simulink model "model_no_heading_control"  (R2023b)
settings: Solver=VariableStepAuto  StartTime=0.0  StopTime=10.0  RelTol=1e-3
values from neighbouring files (symbols this model uses):
  turnrate_ref = 1    [get_heading_tf.m]
  turnrate_ref_start_time = 0.10    (= 0.1)    [get_heading_tf.m]
undefined symbols (not defined in the file or in its folder): acceleration_limit, alpha, D, gear, J, Kb, Ki, Ki_turnrate, Kp, Kp_turnrate, Kt, L, M, R, taud, transport_delay, Ts, turn_acc_limit, vel_ref, vel_ref_start_time, wheel_distance, wrad, wzi
settings Model: Creator=Gianluca  LastModifiedBy=simone

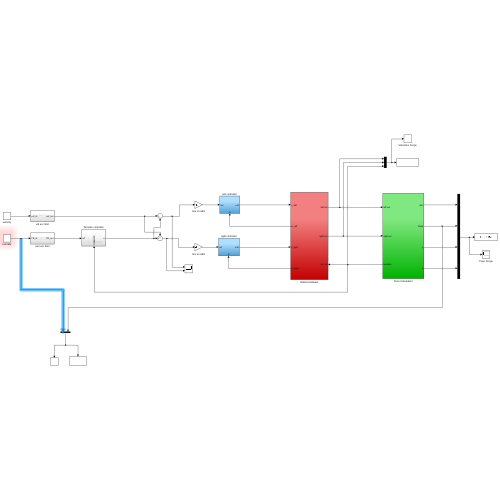
[thumbnail: Simulink's stored preview of the top-level diagram]
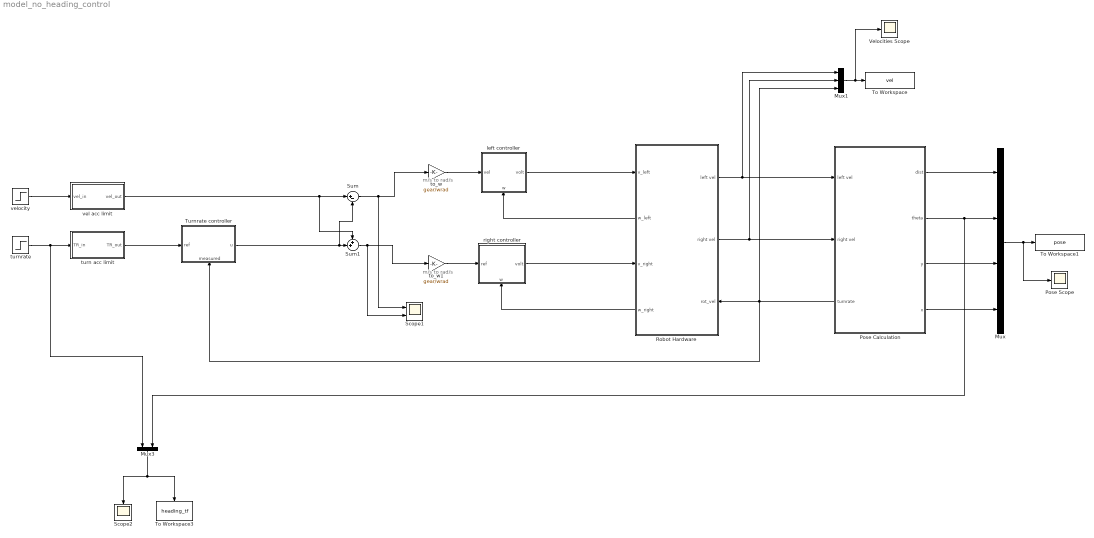
== system model_no_heading_control ==
  note: m/s to rad/s
  note: m/s to rad/s
  Mux : Mux
  Mux1 : Mux  Inputs=3
  Mux3 : Mux  Inputs=2
  Pose Calculation : Subsystem
      settings: PortSchema="{\"entries\":[{\"content\":{\"sides\":[{\"content\":{\"connectorIds\":[\"In1\",\"In2\",\"Out5\"]},\"type\":\"ConnectorPlacement.EquallySpacedRectSide\",\"uuid\":\"3bde791d-a2ac-4d13-a51a-30874ee8f75a\"},{\"content\":{\"connectorIds\":[\"Out1\",\"Out2\",\"Out3\",\"Out4\"],\"side\":\"RIGHT\"},\"type\":\"ConnectorPlacement.EquallySpacedRectSide\",\"uuid\":\"88ae4683-d3e7-483e-be55-3d26372f5fe2\"},{\"content\":{\"side\":\"TOP\"},\"type\":\"ConnectorPlacement.EquallySpacedRectSide\",\"uuid\":\"26752a72-f697-4de9-9dcd-1ca4cee0df39\"}]},\"type\":\"ConnectorPlacement.EquallySpacedConnector\",\"uuid\":\"d259c3e3-c5d7-42b6-881b-3a633aa969c6\"}],\"packageUris\":[\"http://schema.mathworks.com/mf0/Connector/R2020b\"],\"version\":\"1.0\"}"
  Pose Scope : Scope
  Robot Hardware : Subsystem
      settings: PortSchema="{\"entries\":[{\"content\":{\"sides\":[{\"content\":{\"connectorIds\":[\"In1\",\"Out3\",\"In2\",\"Out4\"]},\"type\":\"ConnectorPlacement.EquallySpacedRectSide\",\"uuid\":\"419fea77-f9ca-4e06-bea6-681a18650ab8\"},{\"content\":{\"connectorIds\":[\"Out1\",\"Out2\",\"In3\"],\"side\":\"RIGHT\"},\"type\":\"ConnectorPlacement.EquallySpacedRectSide\",\"uuid\":\"1629cad4-6101-470f-acc1-fad0cb327def\"},{\"content\":{\"side\":\"TOP\"},\"type\":\"ConnectorPlacement.EquallySpacedRectSide\",\"uuid\":\"70c90e71-c188-4b9c-b220-781da08827f9\"}]},\"type\":\"ConnectorPlacement.EquallySpacedConnector\",\"uuid\":\"ad56978f-143c-418e-863d-6c6f1f6f5d0c\"}],\"packageUris\":[\"http://schema.mathworks.com/mf0/Connector/R2020b\"],\"version\":\"1.0\"}"
  Scope1 : Scope  NumInputPorts=2
  Scope2 : Scope
  Sum : Sum  Inputs=|+-
  Sum1 : Sum  Inputs=++|
  To Workspace : ToWorkspace  VariableName=vel  SaveFormat=Timeseries  SampleTime=-1
  To Workspace1 : ToWorkspace  VariableName=pose  SaveFormat=Timeseries  SampleTime=-1
  To Workspace3 : ToWorkspace  VariableName=heading_tf  SaveFormat=Timeseries  SampleTime=-1
  Turnrate controller : Subsystem
      settings: PortSchema="{\"entries\":[{\"content\":{\"sides\":[{\"content\":{\"connectorIds\":[\"In1\"]},\"type\":\"ConnectorPlacement.EquallySpacedRectSide\",\"uuid\":\"3bde791d-a2ac-4d13-a51a-30874ee8f75a\"},{\"content\":{\"connectorIds\":[\"Out1\"],\"side\":\"RIGHT\"},\"type\":\"ConnectorPlacement.EquallySpacedRectSide\",\"uuid\":\"88ae4683-d3e7-483e-be55-3d26372f5fe2\"},{\"content\":{\"side\":\"TOP\"},\"type\":\"ConnectorPlacement.EquallySpacedRectSide\",\"uuid\":\"26752a72-f697-4de9-9dcd-1ca4cee0df39\"},{\"content\":{\"connectorIds\":[\"In2\"],\"side\":\"BOTTOM\"},\"type\":\"ConnectorPlacement.EquallySpacedRectSide\",\"uuid\":\"98a7b674-7c45-4a73-92a3-8750bdde1f36\"}]},\"type\":\"ConnectorPlacement.EquallySpacedConnector\",\"uuid\":\"d259c3e3-c5d7-42b6-881b-3a633aa969c6\"}],\"packageUris\":[\"http://schema.mathworks.com/mf0/Connector/R2020b\"],\"version\":\"1.0\"}"
  Velocities Scope : Scope
  left controller : Subsystem
      settings: PortSchema="{\"entries\":[{\"content\":{\"sides\":[{\"content\":{\"connectorIds\":[\"In1\"]},\"type\":\"ConnectorPlacement.EquallySpacedRectSide\",\"uuid\":\"3bde791d-a2ac-4d13-a51a-30874ee8f75a\"},{\"content\":{\"connectorIds\":[\"Out1\"],\"side\":\"RIGHT\"},\"type\":\"ConnectorPlacement.EquallySpacedRectSide\",\"uuid\":\"88ae4683-d3e7-483e-be55-3d26372f5fe2\"},{\"content\":{\"side\":\"TOP\"},\"type\":\"ConnectorPlacement.EquallySpacedRectSide\",\"uuid\":\"26752a72-f697-4de9-9dcd-1ca4cee0df39\"},{\"content\":{\"connectorIds\":[\"In2\"],\"side\":\"BOTTOM\"},\"type\":\"ConnectorPlacement.EquallySpacedRectSide\",\"uuid\":\"8837b86a-35cd-4679-9975-e69b760c287c\"}]},\"type\":\"ConnectorPlacement.EquallySpacedConnector\",\"uuid\":\"d259c3e3-c5d7-42b6-881b-3a633aa969c6\"}],\"packageUris\":[\"http://schema.mathworks.com/mf0/Connector/R2020b\"],\"version\":\"1.0\"}"
  right controller : Subsystem
      settings: PortSchema="{\"entries\":[{\"content\":{\"sides\":[{\"content\":{\"connectorIds\":[\"In1\"]},\"type\":\"ConnectorPlacement.EquallySpacedRectSide\",\"uuid\":\"3bde791d-a2ac-4d13-a51a-30874ee8f75a\"},{\"content\":{\"connectorIds\":[\"Out1\"],\"side\":\"RIGHT\"},\"type\":\"ConnectorPlacement.EquallySpacedRectSide\",\"uuid\":\"88ae4683-d3e7-483e-be55-3d26372f5fe2\"},{\"content\":{\"side\":\"TOP\"},\"type\":\"ConnectorPlacement.EquallySpacedRectSide\",\"uuid\":\"26752a72-f697-4de9-9dcd-1ca4cee0df39\"},{\"content\":{\"connectorIds\":[\"In2\"],\"side\":\"BOTTOM\"},\"type\":\"ConnectorPlacement.EquallySpacedRectSide\",\"uuid\":\"1adabdfb-f360-4bb8-8b57-8160c74899b3\"}]},\"type\":\"ConnectorPlacement.EquallySpacedConnector\",\"uuid\":\"d259c3e3-c5d7-42b6-881b-3a633aa969c6\"}],\"packageUris\":[\"http://schema.mathworks.com/mf0/Connector/R2020b\"],\"version\":\"1.0\"}"
  to_w : Gain  Gain=gear/wrad
  to_w1 : Gain  Gain=gear/wrad
  turn acc limit : Subsystem
  turnrate : Step  Time=turnrate_ref_start_time  After=turnrate_ref  SampleTime=0
  vel acc limit : Subsystem
  velocity : Step  Time=vel_ref_start_time  After=vel_ref  SampleTime=0
  wires:
  Sum/1 -> Scope1/1, to_w/1
  Sum1/1 -> Scope1/2, to_w1/1
  to_w/1 -> left controller/1(vel)
  to_w1/1 -> right controller/1(ref)
  Robot Hardware/4(w_right) -> right controller/2(w)
  right controller/1(volt) -> Robot Hardware/2(v_right)
  Robot Hardware/3(w_left) -> left controller/2(w)
  left controller/1(volt) -> Robot Hardware/1(v_left)
  Pose Calculation/5(turnrate) -> Turnrate controller/2(measured), Robot Hardware/3(rot_vel), Mux1/3
  Robot Hardware/2(right vel) -> Pose Calculation/2(right vel), Mux1/2
  Robot Hardware/1(left vel) -> Mux1/1, Pose Calculation/1(left vel)
  Mux/1 -> Pose Scope/1, To Workspace1/1
  Pose Calculation/3(y) -> Mux/3
  Pose Calculation/2(theta) -> Mux/2, Mux3/2
  Pose Calculation/1(dist) -> Mux/1
  Pose Calculation/4(x) -> Mux/4
  Mux1/1 -> Velocities Scope/1, To Workspace/1
  Turnrate controller/1(u) -> Sum/2, Sum1/2
  velocity/1 -> vel acc limit/1(vel_in)
  turnrate/1 -> Mux3/1, turn acc limit/1(TR_in)
  Mux3/1 -> To Workspace3/1, Scope2/1
  turn acc limit/1(TR_out) -> Turnrate controller/1(ref)
  vel acc limit/1(vel_out) -> Sum1/1, Sum/1

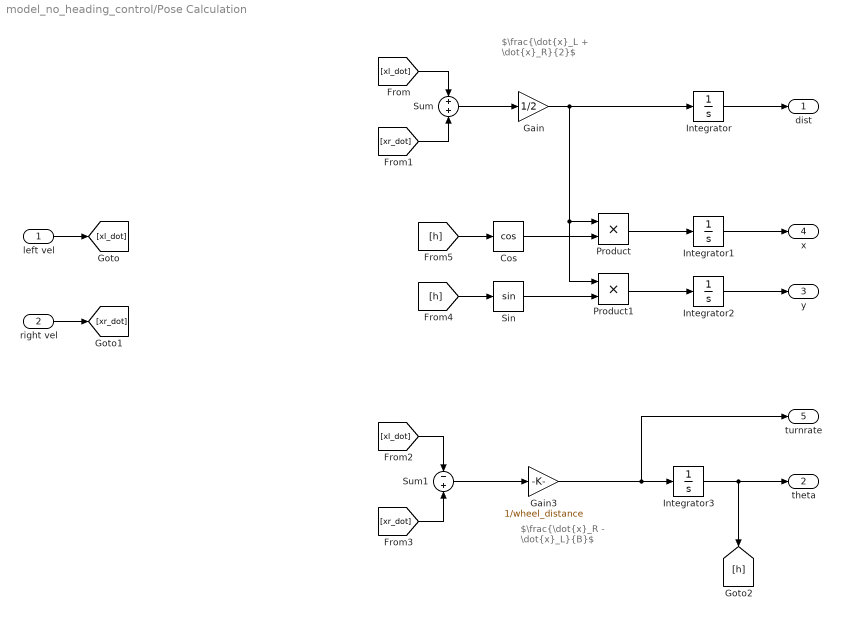
== system model_no_heading_control/Pose Calculation ==
  note: $\frac{\dot{x}_L + \dot{x}_R}{2}$
  note: $\frac{\dot{x}_R - \dot{x}_L}{B}$
  left vel : Inport
  right vel : Inport  Port=2
  Cos : Trigonometry  Operator=cos
  Gain : Gain  Gain=1/2
  Gain3 : Gain  Gain=1/wheel_distance
  Integrator{,1..3} (4 alike) : Integrator
  Product : Product
  Product1 : Product
  Sin : Trigonometry
  Sum : Sum  Inputs=+|+
  Sum1 : Sum  Inputs=-|+
  dist : Outport
  theta : Outport  Port=2
  y : Outport  Port=3
  x : Outport  Port=4
  turnrate : Outport  Port=5
  wires:
  Sum/1 -> Gain/1
  Gain/1 -> Integrator/1, Product/1, Product1/1
  Integrator/1 -> dist/1
  left vel/1 -> [xl_dot]
  right vel/1 -> [xr_dot]
  [xl_dot] -> Sum/1
  [xr_dot] -> Sum/2
  [xl_dot] -> Sum1/1
  [xr_dot] -> Sum1/2
  Gain3/1 -> turnrate/1, Integrator3/1
  Sum1/1 -> Gain3/1
  Integrator3/1 -> theta/1, [h]
  [h] -> Sin/1
  Integrator2/1 -> y/1
  Integrator1/1 -> x/1
  [h] -> Cos/1
  Sin/1 -> Product1/2
  Cos/1 -> Product/2
  Product1/1 -> Integrator2/1
  Product/1 -> Integrator1/1

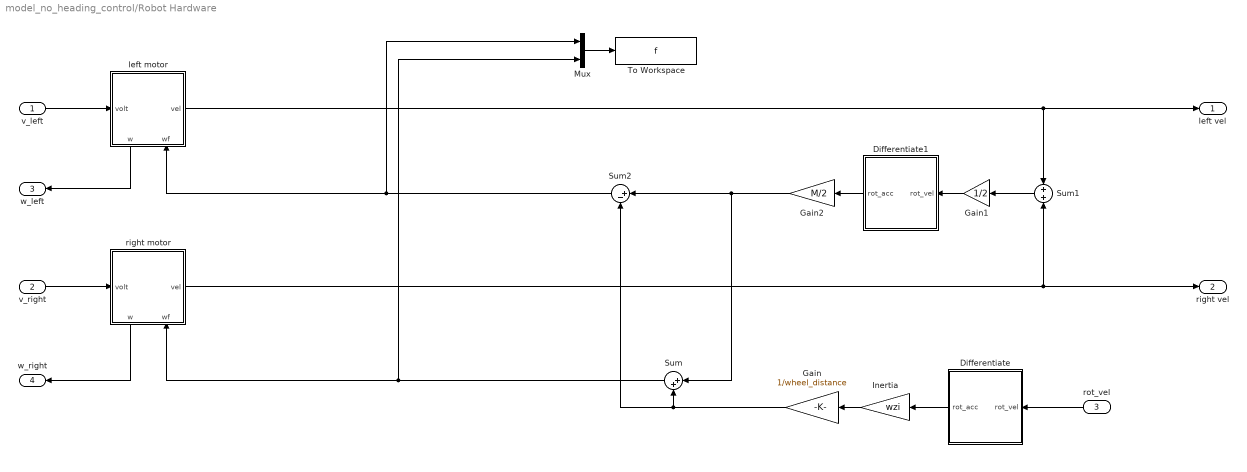
== system model_no_heading_control/Robot Hardware ==
  v_left : Inport
  v_right : Inport  Port=2
  rot_vel : Inport  Port=3
  Differentiate : Subsystem
  Differentiate1 : Subsystem
  Gain : Gain  Gain=1/wheel_distance
  Gain1 : Gain  Gain=1/2
  Gain2 : Gain  Gain=M/2
  Inertia : Gain  Gain=wzi
  Mux : Mux  Inputs=2
  Sum : Sum  Inputs=|++
  Sum1 : Sum  Inputs=+|+
  Sum2 : Sum  Inputs=|+-
  To Workspace : ToWorkspace  VariableName=f  SaveFormat=Timeseries  SampleTime=-1
  left motor : Subsystem
      settings: PortSchema="{\"entries\":[{\"content\":{\"sides\":[{\"content\":{\"connectorIds\":[\"In1\"]},\"type\":\"ConnectorPlacement.EquallySpacedRectSide\",\"uuid\":\"3bde791d-a2ac-4d13-a51a-30874ee8f75a\"},{\"content\":{\"connectorIds\":[\"Out1\"],\"side\":\"RIGHT\"},\"type\":\"ConnectorPlacement.EquallySpacedRectSide\",\"uuid\":\"88ae4683-d3e7-483e-be55-3d26372f5fe2\"},{\"content\":{\"side\":\"TOP\"},\"type\":\"ConnectorPlacement.EquallySpacedRectSide\",\"uuid\":\"26752a72-f697-4de9-9dcd-1ca4cee0df39\"},{\"content\":{\"connectorIds\":[\"Out2\",\"In2\"],\"side\":\"BOTTOM\"},\"type\":\"ConnectorPlacement.EquallySpacedRectSide\",\"uuid\":\"bdf58d17-97a4-48aa-9393-076eaaeca649\"}]},\"type\":\"ConnectorPlacement.EquallySpacedConnector\",\"uuid\":\"d259c3e3-c5d7-42b6-881b-3a633aa969c6\"}],\"packageUris\":[\"http://schema.mathworks.com/mf0/Connector/R2020b\"],\"version\":\"1.0\"}"
  right motor : Subsystem
      settings: PortSchema="{\"entries\":[{\"content\":{\"sides\":[{\"content\":{\"connectorIds\":[\"In1\"]},\"type\":\"ConnectorPlacement.EquallySpacedRectSide\",\"uuid\":\"3bde791d-a2ac-4d13-a51a-30874ee8f75a\"},{\"content\":{\"connectorIds\":[\"Out1\"],\"side\":\"RIGHT\"},\"type\":\"ConnectorPlacement.EquallySpacedRectSide\",\"uuid\":\"88ae4683-d3e7-483e-be55-3d26372f5fe2\"},{\"content\":{\"side\":\"TOP\"},\"type\":\"ConnectorPlacement.EquallySpacedRectSide\",\"uuid\":\"26752a72-f697-4de9-9dcd-1ca4cee0df39\"},{\"content\":{\"connectorIds\":[\"Out2\",\"In2\"],\"side\":\"BOTTOM\"},\"type\":\"ConnectorPlacement.EquallySpacedRectSide\",\"uuid\":\"bdf58d17-97a4-48aa-9393-076eaaeca649\"}]},\"type\":\"ConnectorPlacement.EquallySpacedConnector\",\"uuid\":\"d259c3e3-c5d7-42b6-881b-3a633aa969c6\"}],\"packageUris\":[\"http://schema.mathworks.com/mf0/Connector/R2020b\"],\"version\":\"1.0\"}"
  left vel : Outport
  right vel : Outport  Port=2
  w_left : Outport  Port=3
  w_right : Outport  Port=4
  wires:
  v_left/1 -> left motor/1(volt)
  left motor/2(w) -> w_left/1
  v_right/1 -> right motor/1(volt)
  right motor/2(w) -> w_right/1
  Mux/1 -> To Workspace/1
  rot_vel/1 -> Differentiate/1(rot_vel)
  Differentiate/1(rot_acc) -> Inertia/1
  Inertia/1 -> Gain/1
  Gain/1 -> Sum/2, Sum2/2
  Sum/1 -> right motor/2(wf), Mux/2
  left motor/1(vel) -> Sum1/1, left vel/1
  Sum1/1 -> Gain1/1
  Gain1/1 -> Differentiate1/1(rot_vel)
  Differentiate1/1(rot_acc) -> Gain2/1
  Gain2/1 -> Sum/1, Sum2/1
  Sum2/1 -> left motor/2(wf), Mux/1
  right motor/1(vel) -> Sum1/2, right vel/1

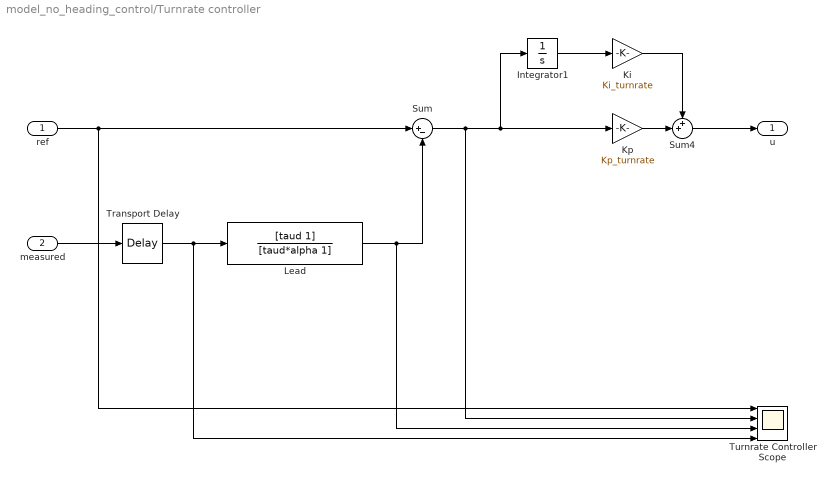
== system model_no_heading_control/Turnrate controller ==
  ref : Inport
  measured : Inport  Port=2
  Integrator1 : Integrator
  Ki : Gain  Gain=Ki_turnrate
  Kp : Gain  Gain=Kp_turnrate
  Lead : TransferFcn  Numerator=[taud 1]  Denominator=[taud*alpha 1]
  Sum : Sum  Inputs=|+-
  Sum4 : Sum  Inputs=++|
  Transport Delay : TransportDelay  DelayTime=transport_delay
  Turnrate Controller Scope : Scope  NumInputPorts=4
  u : Outport
  wires:
  ref/1 -> Turnrate Controller Scope/1, Sum/1
  Lead/1 -> Sum/2, Turnrate Controller Scope/3
  measured/1 -> Transport Delay/1
  Transport Delay/1 -> Turnrate Controller Scope/4, Lead/1
  Sum4/1 -> u/1
  Sum/1 -> Turnrate Controller Scope/2, Integrator1/1, Kp/1
  Integrator1/1 -> Ki/1
  Ki/1 -> Sum4/1
  Kp/1 -> Sum4/2

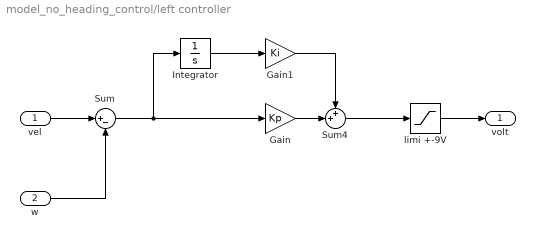
== system model_no_heading_control/left controller ==
  vel : Inport
  w : Inport  Port=2
  Gain : Gain  Gain=Kp
  Gain1 : Gain  Gain=Ki
  Integrator : Integrator
  Sum : Sum  Inputs=|+-
  Sum4 : Sum  Inputs=++|
  limi +-9V : Saturate  UpperLimit=9  LowerLimit=-9
  volt : Outport
  wires:
  Gain/1 -> Sum4/2
  Integrator/1 -> Gain1/1
  Gain1/1 -> Sum4/1
  vel/1 -> Sum/1
  w/1 -> Sum/2
  Sum/1 -> Integrator/1, Gain/1
  Sum4/1 -> limi +-9V/1
  limi +-9V/1 -> volt/1

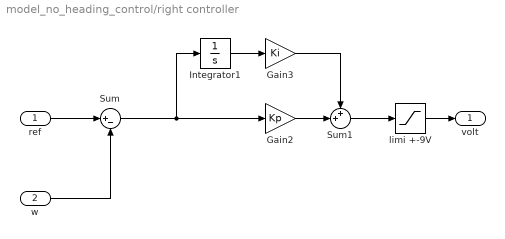
== system model_no_heading_control/right controller ==
  ref : Inport
  w : Inport  Port=2
  Gain2 : Gain  Gain=Kp
  Gain3 : Gain  Gain=Ki
  Integrator1 : Integrator
  Sum : Sum  Inputs=|+-
  Sum1 : Sum  Inputs=++|
  limi +-9V : Saturate  UpperLimit=9  LowerLimit=-9
  volt : Outport
  wires:
  Integrator1/1 -> Gain3/1
  Gain2/1 -> Sum1/2
  Gain3/1 -> Sum1/1
  Sum/1 -> Integrator1/1, Gain2/1
  ref/1 -> Sum/1
  w/1 -> Sum/2
  Sum1/1 -> limi +-9V/1
  limi +-9V/1 -> volt/1

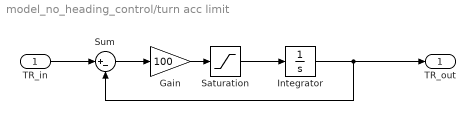
== system model_no_heading_control/turn acc limit ==
  TR_in : Inport
  Gain : Gain  Gain=100
  Integrator : Integrator
  Saturation : Saturate  UpperLimit=turn_acc_limit  LowerLimit=-turn_acc_limit
  Sum : Sum  Inputs=|+-
  TR_out : Outport
  wires:
  TR_in/1 -> Sum/1
  Sum/1 -> Gain/1
  Gain/1 -> Saturation/1
  Saturation/1 -> Integrator/1
  Integrator/1 -> Sum/2, TR_out/1

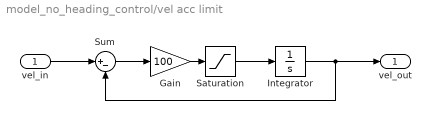
== system model_no_heading_control/vel acc limit ==
  vel_in : Inport
  Gain : Gain  Gain=100
  Integrator : Integrator
  Saturation : Saturate  UpperLimit=acceleration_limit  LowerLimit=-acceleration_limit
  Sum : Sum  Inputs=|+-
  vel_out : Outport
  wires:
  vel_in/1 -> Sum/1
  Sum/1 -> Gain/1
  Gain/1 -> Saturation/1
  Saturation/1 -> Integrator/1
  Integrator/1 -> Sum/2, vel_out/1

== system model_no_heading_control/Robot Hardware/Differentiate ==
  rot_vel : Inport
  Gain : Gain  Gain=100
  Integrator : Integrator
  Sum : Sum  Inputs=|+-
  rot_acc : Outport
  wires:
  rot_vel/1 -> Sum/1
  Sum/1 -> Gain/1
  Integrator/1 -> Sum/2
  Gain/1 -> rot_acc/1, Integrator/1

== system model_no_heading_control/Robot Hardware/Differentiate1 ==
  rot_vel : Inport
  Gain : Gain  Gain=100
  Integrator : Integrator
  Sum : Sum  Inputs=|+-
  rot_acc : Outport
  wires:
  rot_vel/1 -> Sum/1
  Sum/1 -> Gain/1
  Integrator/1 -> Sum/2
  Gain/1 -> rot_acc/1, Integrator/1

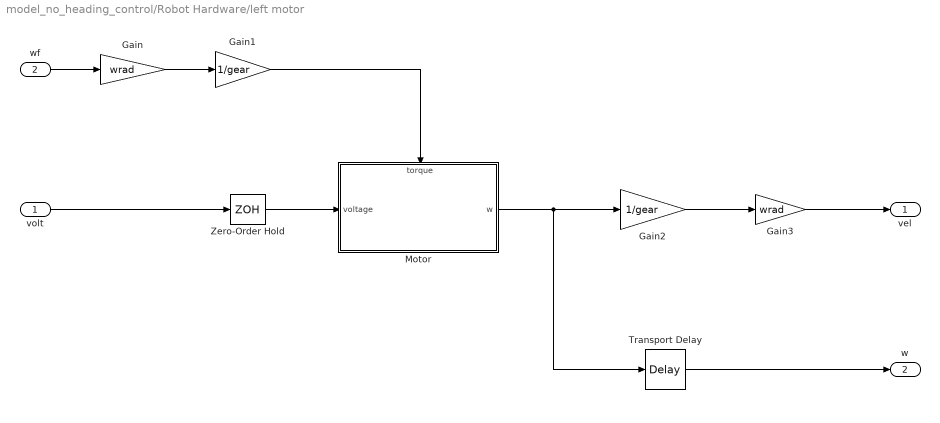
== system model_no_heading_control/Robot Hardware/left motor ==
  volt : Inport
  wf : Inport  Port=2
  Gain : Gain  Gain=wrad
  Gain1 : Gain  Gain=1/gear
  Gain2 : Gain  Gain=1/gear
  Gain3 : Gain  Gain=wrad
  Motor : Subsystem
      settings: PortSchema="{\"entries\":[{\"content\":{\"sides\":[{\"content\":{\"connectorIds\":[\"In1\"]},\"type\":\"ConnectorPlacement.EquallySpacedRectSide\",\"uuid\":\"3bde791d-a2ac-4d13-a51a-30874ee8f75a\"},{\"content\":{\"connectorIds\":[\"Out1\"],\"side\":\"RIGHT\"},\"type\":\"ConnectorPlacement.EquallySpacedRectSide\",\"uuid\":\"88ae4683-d3e7-483e-be55-3d26372f5fe2\"},{\"content\":{\"connectorIds\":[\"In2\"],\"side\":\"TOP\"},\"type\":\"ConnectorPlacement.EquallySpacedRectSide\",\"uuid\":\"26752a72-f697-4de9-9dcd-1ca4cee0df39\"}]},\"type\":\"ConnectorPlacement.EquallySpacedConnector\",\"uuid\":\"d259c3e3-c5d7-42b6-881b-3a633aa969c6\"}],\"packageUris\":[\"http://schema.mathworks.com/mf0/Connector/R2020b\"],\"version\":\"1.0\"}"
  Transport Delay : TransportDelay  DelayTime=transport_delay
  Zero-Order Hold : ZeroOrderHold  SampleTime=Ts
  vel : Outport
  w : Outport  Port=2
  wires:
  wf/1 -> Gain/1
  Gain/1 -> Gain1/1
  Gain1/1 -> Motor/2(torque)
  Gain3/1 -> vel/1
  Gain2/1 -> Gain3/1
  Motor/1(w) -> Transport Delay/1, Gain2/1
  Transport Delay/1 -> w/1
  volt/1 -> Zero-Order Hold/1
  Zero-Order Hold/1 -> Motor/1(voltage)

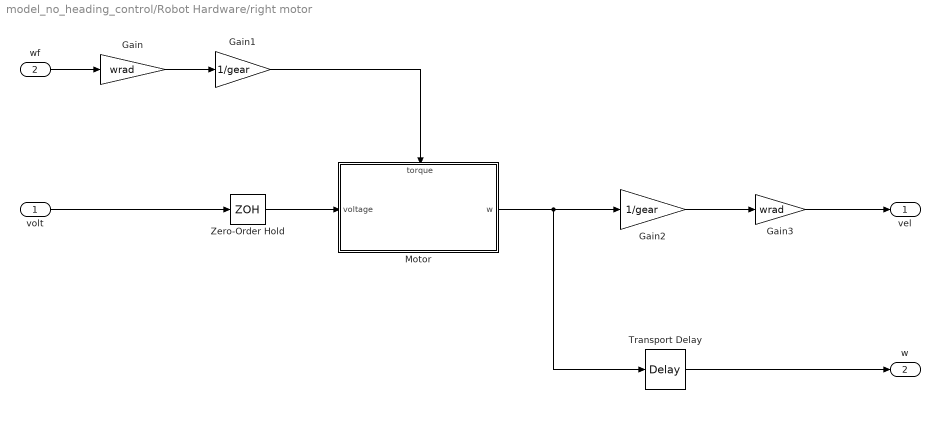
== system model_no_heading_control/Robot Hardware/right motor ==
  volt : Inport
  wf : Inport  Port=2
  Gain : Gain  Gain=wrad
  Gain1 : Gain  Gain=1/gear
  Gain2 : Gain  Gain=1/gear
  Gain3 : Gain  Gain=wrad
  Motor : Subsystem
      settings: PortSchema="{\"entries\":[{\"content\":{\"sides\":[{\"content\":{\"connectorIds\":[\"In1\"]},\"type\":\"ConnectorPlacement.EquallySpacedRectSide\",\"uuid\":\"3bde791d-a2ac-4d13-a51a-30874ee8f75a\"},{\"content\":{\"connectorIds\":[\"Out1\"],\"side\":\"RIGHT\"},\"type\":\"ConnectorPlacement.EquallySpacedRectSide\",\"uuid\":\"88ae4683-d3e7-483e-be55-3d26372f5fe2\"},{\"content\":{\"connectorIds\":[\"In2\"],\"side\":\"TOP\"},\"type\":\"ConnectorPlacement.EquallySpacedRectSide\",\"uuid\":\"26752a72-f697-4de9-9dcd-1ca4cee0df39\"}]},\"type\":\"ConnectorPlacement.EquallySpacedConnector\",\"uuid\":\"d259c3e3-c5d7-42b6-881b-3a633aa969c6\"}],\"packageUris\":[\"http://schema.mathworks.com/mf0/Connector/R2020b\"],\"version\":\"1.0\"}"
  Transport Delay : TransportDelay  DelayTime=transport_delay
  Zero-Order Hold : ZeroOrderHold  SampleTime=Ts
  vel : Outport
  w : Outport  Port=2
  wires:
  wf/1 -> Gain/1
  Gain/1 -> Gain1/1
  Gain1/1 -> Motor/2(torque)
  Gain3/1 -> vel/1
  Gain2/1 -> Gain3/1
  Motor/1(w) -> Transport Delay/1, Gain2/1
  Transport Delay/1 -> w/1
  volt/1 -> Zero-Order Hold/1
  Zero-Order Hold/1 -> Motor/1(voltage)

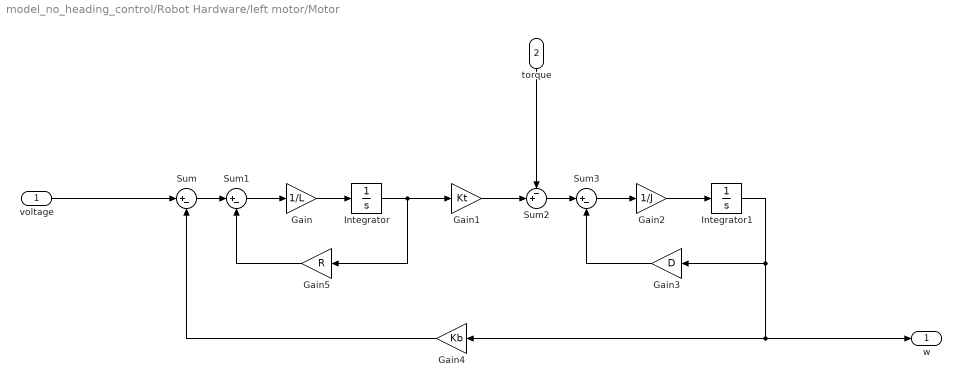
== system model_no_heading_control/Robot Hardware/left motor/Motor ==
  voltage : Inport
  torque : Inport  Port=2
  Gain : Gain  Gain=1/L
  Gain1 : Gain  Gain=Kt
  Gain2 : Gain  Gain=1/J
  Gain3 : Gain  Gain=D
  Gain4 : Gain  Gain=Kb
  Gain5 : Gain  Gain=R
  Integrator : Integrator
  Integrator1 : Integrator
  Sum : Sum  Inputs=|+-
  Sum1 : Sum  Inputs=|+-
  Sum2 : Sum  Inputs=-+|
  Sum3 : Sum  Inputs=|+-
  w : Outport
  wires:
  voltage/1 -> Sum/1
  Sum/1 -> Sum1/1
  Gain/1 -> Integrator/1
  Gain1/1 -> Sum2/2
  Integrator/1 -> Gain5/1, Gain1/1
  torque/1 -> Sum2/1
  Sum2/1 -> Sum3/1
  Sum3/1 -> Gain2/1
  Gain2/1 -> Integrator1/1
  Integrator1/1 -> Gain3/1, Gain4/1, w/1
  Gain3/1 -> Sum3/2
  Gain4/1 -> Sum/2
  Gain5/1 -> Sum1/2
  Sum1/1 -> Gain/1

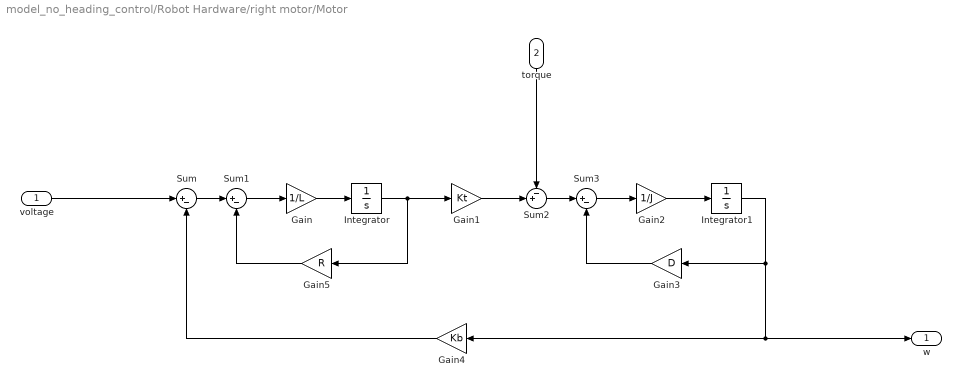
== system model_no_heading_control/Robot Hardware/right motor/Motor ==
  voltage : Inport
  torque : Inport  Port=2
  Gain : Gain  Gain=1/L
  Gain1 : Gain  Gain=Kt
  Gain2 : Gain  Gain=1/J
  Gain3 : Gain  Gain=D
  Gain4 : Gain  Gain=Kb
  Gain5 : Gain  Gain=R
  Integrator : Integrator
  Integrator1 : Integrator
  Sum : Sum  Inputs=|+-
  Sum1 : Sum  Inputs=|+-
  Sum2 : Sum  Inputs=-+|
  Sum3 : Sum  Inputs=|+-
  w : Outport
  wires:
  voltage/1 -> Sum/1
  Sum/1 -> Sum1/1
  Gain/1 -> Integrator/1
  Gain1/1 -> Sum2/2
  Integrator/1 -> Gain5/1, Gain1/1
  torque/1 -> Sum2/1
  Sum2/1 -> Sum3/1
  Sum3/1 -> Gain2/1
  Gain2/1 -> Integrator1/1
  Integrator1/1 -> Gain3/1, Gain4/1, w/1
  Gain3/1 -> Sum3/2
  Gain4/1 -> Sum/2
  Gain5/1 -> Sum1/2
  Sum1/1 -> Gain/1
